simulink model "Flowchart10"  (Simulink 6.0)
settings: Solver=FixedStepDiscrete  StartTime=0.0  StopTime=10.0  RelTol=1e-3
settings Model: Creator=scaife  LastModifiedBy=scaife  ExtModeAutoUpdateStatusClock=off
settings DataIOCC: SignalLoggingName=sigsOut
settings DebuggingCC: SolverPrmCheckMsg=none
settings HardwareCC: TargetUnknown=on
settings STFCustomTargetCC: TargetFcnLib=ansi_tfl_tmw.mat  GenFloatMathFcnCalls=ANSI_C  ModelReferenceCompliant=off  SystemTargetFile=grt.tlc

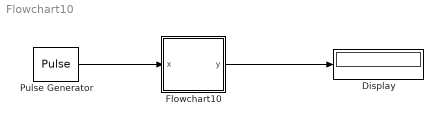
== system Flowchart10 ==
  Display : Display
  Flowchart10 : Stateflow chart
  Pulse Generator : DiscretePulseGenerator
  wires:
  Pulse Generator/1 -> Flowchart10/1(x)
  Flowchart10/1(y) -> Display/1

== stateflow chart Flowchart10 ==
  state A [parallel]
    (default) -> (junction 4) : [x==0]{y++;}
    (default) -> (junction 5) : [x>0]{y--;}
    A -> (junction 6) : [x>0]{y-=2;}
    A -> (junction 7) : [x==0]{y+=2;}
  data: x input int32; y output int32
